simulink model "ACC_speed_change_curve_cs"  (R2016a)
settings: Solver=ode5  SolverMode=SingleTasking  StartTime=0.0  StopTime=inf  FixedStep=1/1000  RelTol=1e-3
PreLoadFcn:
  | mbxruntime.callbacks.PreLoadFcn(bdroot);
  | check_NUTS_defined;
  | 
  | assignin('base',['model_closed_' bdroot],false);addpath('../includes_ACC');
PostLoadFcn:
  | mbxruntime.callbacks.PostLoadFcn(bdroot);
InitFcn:
  | mbxruntime.callbacks.InitFcn(bdroot);
StartFcn:
  | mbxruntime.callbacks.StartFcn(bdroot);
StopFcn:
  | mbxruntime.callbacks.StopFcn(bdroot);
model workspace (MAT data in the model file):
  mbox_table : struct (value not decoded)
  model_closed = 0
  sim_status = 0
undefined symbols (not defined in the file or in its folder): DiscIntNeverNeededParam
undefined symbols (not defined in the file): SteeringColumn, SteeringWheel, WheelL0, WheelL1, WheelR0, WheelR1
libraries: simulink_extras x49, simulink x29, PreScanSimulinkLibrary x24, PreScanUsefulBlocks x2, Solver_SF x1, simulink_need_slupdate x1
(part 10 of 17)

== system ACC_speed_change_curve_cs/Audi_A8_1/ACC_System/TIS2 Straight Road ==
  note: === TIS2 Straight Road block ===
      |
      |  - interpretes information provided from the second TIS sensor,
      |  - computes HeadWay Time (HWT) for object on the lane in front of the EGO car,
      |  - determines if detected objects is potentially dengerous,
      |  - outputs distance to the following car, computes its velocity and safe distance to be kept.
  EGO_velocity [m/s] : Inport
  TIS2_range [m] : Inport  Port=2  PortDimensions=TISdet(2)
  TIS2_rangedot [m/s] : Inport  Port=3  PortDimensions=TISdet(2)
  TIS2_theta [deg] : Inport  Port=4  PortDimensions=TISdet(2)
  HWT_dem [s] : Inport  Port=5
  Standstill [m] : Inport  Port=6
  HWT_dem [s]1 : InportShadow  Port=5
  Hold : Subsystem
  TIS2 Closest Object : Subsystem
  TIS2 HWT Computing : Subsystem
  TIS2 HWT Computing2 : Subsystem
  TIS2 HWT Flag : Subsystem
  TIS2 Lead Car Longitudinal Velocity : Subsystem
  TIS2 Objects On Lane : Subsystem
  TIS2 Sorting Fun : Subsystem
  TIS2_closest_object_search : MATLAB Function  TreatAsAtomicUnit=on
  HWT_flag : Outport
  TIS2 Lead distance [m] : Outport  Port=2
  TIS2 Safe_distance [m] : Outport  Port=3
  TIS2_HWT_straight : Outport  Port=4
  TIS2 Lead velocity [m/s] : Outport  Port=5
  index : Outport  Port=6
  wires:
  TIS2 Lead Car Longitudinal Velocity/1(Safe distance [m]) -> TIS2 Safe_distance [m]/1
  HWT_dem [s]/1 -> TIS2 Lead Car Longitudinal Velocity/1(HWT_dem (s)), TIS2 HWT Flag/2(HWT_dem [s])
  TIS2 Closest Object/1(rangedot [m/s]) -> TIS2 Lead Car Longitudinal Velocity/2(TIS2 Rangedot [m/s])
  TIS2 Closest Object/2(distance [m/s]) -> TIS2 Lead distance [m]/1, TIS2 HWT Computing2/1(Distance [m]), TIS2 HWT Flag/1(Distance closest [m])
  EGO_velocity [m/s]/1 -> TIS2 Lead Car Longitudinal Velocity/3(EGO Velocity [m/s]), TIS2 HWT Computing2/2(Velocity [m/s]), TIS2 HWT Computing/3(Velocity [m/s])
  TIS2 HWT Computing/1(HWT [s]) -> TIS2 HWT Flag/3(HWT [s])
  TIS2_closest_object_search/1(index) -> TIS2 Closest Object/3(index), index/1
  TIS2 Sorting Fun/3(TIS2_THETA [rad]) -> TIS2 Objects On Lane/3(TIS2_theta [rad])
  TIS2 Sorting Fun/2(TIS2_RANGEDOT [m/s]) -> TIS2 Objects On Lane/2(TIS2_rangedot [m/s])
  TIS2 Sorting Fun/1(TIS2_RANGE [m]) -> TIS2 Objects On Lane/1(TIS2_range [m])
  TIS2_theta [deg]/1 -> TIS2 Sorting Fun/3(TIS2theta [deg])
  TIS2_rangedot [m/s]/1 -> TIS2 Sorting Fun/2(TIS2rangedot [m/s])
  TIS2_range [m]/1 -> TIS2 Sorting Fun/1(TIS2range [m])
  Standstill [m]/1 -> TIS2 Lead Car Longitudinal Velocity/4(Standstill [m]), TIS2 HWT Flag/4(Standstill distance)
  TIS2 Objects On Lane/1(TIS2_RANGEDOT [m/s]) -> TIS2 Closest Object/1(TIS2_rangedot [m/s])
  TIS2 Lead Car Longitudinal Velocity/2(Lead velocity [m/s]) -> TIS2 Lead velocity [m/s]/1, Hold/2(lead_vel_in)
  TIS2 HWT Computing2/1(HWT [s]) -> TIS2_HWT_straight/1
  TIS2 HWT Flag/1(HWT_flag) -> Hold/1(HWTflagIN)
  Hold/1(HWT_flag) -> HWT_flag/1
  HWT_dem [s]1/1 -> TIS2 HWT Computing/2(HWT demanded)
  TIS2 Objects On Lane/2(TIS2_Distance [m]) -> TIS2 Closest Object/2(TIS2_distance [m]), TIS2_closest_object_search/1(distance), TIS2 HWT Computing/1(Distance [m])

== system ACC_speed_change_curve_cs/Audi_A8_1/ACC_System3/Display ==
  HWT_% : Inport
  ACC_flag : Inport  Port=2
  Lead_car_velocity_[m/s] : Inport  Port=3
  RPM : Inport  Port=4
  EGO Velocity [m/s] : Inport  Port=5
  Brake_Pressure_[bar] : Inport  Port=6
  Throttle_[%] : Inport  Port=7
  Display switch : Constant  Value=DisplaySwitch
  If : If
  If Action Subsystem : Subsystem  TreatAsAtomicUnit=on
  If Action Subsystem1 : Subsystem  TreatAsAtomicUnit=on
  Merge : Merge  InitialOutput=1
  Rate Transition : RateTransition  Integrity=off  OutPortSampleTime=Tsensor
  Rate Transition{1..6,8} (7 alike) : RateTransition  Integrity=off  OutPortSampleTime=1/DisplayFreq
  "GUI_System ON {1} / OFF {0}" : Outport
  wires:
  Rate Transition/1 -> "GUI_System ON {1} / OFF {0}"/1
  Merge/1 -> Rate Transition/1
  If/2 -> If Action Subsystem1/Action
  If Action Subsystem1/1(Out1) -> Merge/2
  If Action Subsystem/1("GUI_System ON {1} / OFF {0}1") -> Merge/1
  If/1 -> If Action Subsystem/Action
  Rate Transition8/1 -> If Action Subsystem/7(Throttle_[%]1)
  Rate Transition6/1 -> If Action Subsystem/6(Lead_car_velocity_[m/s]1)
  Rate Transition5/1 -> If Action Subsystem/5(ACC_flag1)
  Rate Transition4/1 -> If Action Subsystem/4(HWT_%1)
  Rate Transition3/1 -> If Action Subsystem/3(Brake_Pressure_[bar]1)
  Rate Transition2/1 -> If Action Subsystem/2(EGO Velocity [m/s]1)
  Rate Transition1/1 -> If Action Subsystem/1(RPM1)
  Display switch/1 -> If/1
  Throttle_[%]/1 -> Rate Transition8/1
  Lead_car_velocity_[m/s]/1 -> Rate Transition6/1
  ACC_flag/1 -> Rate Transition5/1
  HWT_%/1 -> Rate Transition4/1
  Brake_Pressure_[bar]/1 -> Rate Transition3/1
  EGO Velocity [m/s]/1 -> Rate Transition2/1
  RPM/1 -> Rate Transition1/1

== system ACC_speed_change_curve_cs/Audi_A8_1/ACC_System3/HWT_percentage ==
  TIS1_HWT : Inport
  TIS2_HWT : Inport  Port=2  SampleTime=Tsensor
  HWT_dem_[s] : Inport  Port=3  SampleTime=Tsensor
  Bias : Bias  Bias=-1
  Brake Pressure [ar]1 : Gain  Gain=100
  Constant : Constant  Value=10
  Constant1 : Constant  Value=0
  Demux : Demux  Outputs=2
  Divide : Product  Inputs=*/
  Logical Operator : Logic  AllPortsSameDT=off  OutDataTypeStr=boolean
  Mux : Mux  Inputs=2
  Relational Operator : RelationalOperator  Operator=<  OutDataTypeStr=boolean
  Relational Operator1 : RelationalOperator  Operator=>  OutDataTypeStr=boolean
  TIS1_HWT_perc : Outport
  TIS2_HWT_perc : Outport  Port=2
  wires:
  Constant1/1 -> Relational Operator1/2
  Relational Operator1/1 -> Logical Operator/2
  Logical Operator/1 -> Demux/1
  Relational Operator/1 -> Logical Operator/1
  Demux/2 -> TIS2_HWT_perc/1
  Demux/1 -> TIS1_HWT_perc/1
  HWT_dem_[s]/1 -> Divide/2
  Mux/1 -> Relational Operator1/1, Divide/1
  Constant/1 -> Relational Operator/2
  Brake Pressure [ar]1/1 -> Relational Operator/1
  TIS2_HWT/1 -> Mux/2
  TIS1_HWT/1 -> Mux/1
  Bias/1 -> Brake Pressure [ar]1/1
  Divide/1 -> Bias/1

== system ACC_speed_change_curve_cs/Audi_A8_1/ACC_System3/Limitations1 ==
  note: === Limitations block ===
      |
      |  - switching the system on or off due to the drivers decision,
      |  - limits maximum operating velocity
      |    above which the sensors are becoming ineffective.
  note: if equal to 1 => ACC should be off
      | if equal to 0 => ACC should be on
  Throttle [%] : Inport
  Brake_Pres [bar] : Inport  Port=2
  ACC_flag : Inport  Port=3
  HWT [s] : Inport  Port=4
  Lead car vel : Inport  Port=5
  indx : Inport  Port=6
  "Switch ON {1} / OFF {0}" : Inport  Port=7
  EGO Velocity [m/s] : Inport  Port=8
  Indicator flag : Inport  Port=9
  Throttle_in [%] : Inport  Port=10
  Brake_Pres_in [bar] : Inport  Port=11
  HWT_dem_[s] : Inport  Port=12
  TIS2_Flag : Inport  Port=13
  Compare To Zero : simulink/Logic and Bit Operations/Compare To Zero  relop===  OutDataTypeStr=boolean
  Compare To Zero1 : simulink/Logic and Bit Operations/Compare To Zero  relop=~=  OutDataTypeStr=boolean
  Const : Constant  Value=BrakePressureMax/100
  Constant : Constant  Value=TISdet (2)
  Constant1 : Constant  Value=TISdet (1)
  Gain : Gain  Gain=2
  Gain1 : Gain
  Gain2 : Gain
  Logical Operator : Logic  Operator=OR  Inputs=3  AllPortsSameDT=off  OutDataTypeStr=boolean
  Logical Operator1 : Logic  Operator=OR  AllPortsSameDT=off  OutDataTypeStr=boolean
  MAX Speed [m/s] : Constant  Value=MaxSpeed/3.6
  Rate Limiter : RateLimiter  RisingSlewLimit=BrakePressureMax  FallingSlewLimit=-BrakePressureMax  SampleTimeMode=inherited
  Rate Transition : RateTransition  Integrity=off  OutPortSampleTime=Tsensor
  Relational Operator : RelationalOperator  Operator=>  OutDataTypeStr=boolean
  Relational Operator1 : RelationalOperator  OutDataTypeStr=boolean
  Relational Operator2 : RelationalOperator  Operator===  OutDataTypeStr=boolean
  Saturation Dynamic : simulink/Discontinuities/Saturation Dynamic  OutMin=[]  OutMax=[]  OutDataTypeStr=Inherit: Same as second input  OutDataType=fixdt(1, 16)  OutScaling=2^-10  DoSatur=off
  Switch{,1..6} (7 alike) : Switch  Criteria=u2 > Threshold
  Switch7 : Switch  Criteria=u2 ~= 0
  Zero : Constant  Value=0
  Zero1 : Constant  Value=0
  cond : Subsystem
  Throttle_out [%] : Outport
  Brake_Pres_out [bar] : Outport  Port=2
  ACC flag : Outport  Port=3
  HWT_[s] : Outport  Port=4
  Lead car velocity [m/s] : Outport  Port=5
  wires:
  Rate Limiter/1 -> Switch7/1
  Switch/1 -> Rate Limiter/1, Switch7/3
  Switch7/1 -> Switch4/1, Relational Operator1/1
  cond/1(Out1) -> Switch7/2
  Brake_Pres [bar]/1 -> Switch/3
  Brake_Pres_in [bar]/1 -> Switch/1
  Relational Operator2/1 -> Logical Operator1/2
  Constant1/1 -> Switch6/3
  Constant/1 -> Switch6/1
  Switch6/1 -> Relational Operator2/1
  TIS2_Flag/1 -> Switch6/2
  Rate Transition/1 -> Logical Operator1/1
  Switch4/1 -> Brake_Pres_out [bar]/1
  Zero1/1 -> Switch4/3
  Relational Operator1/1 -> Switch4/2
  Const/1 -> Relational Operator1/2
  Saturation Dynamic/1 -> HWT_[s]/1
  Switch3/1 -> Saturation Dynamic/2
  HWT [s]/1 -> Switch3/3
  Logical Operator1/1 -> Switch3/2
  indx/1 -> Relational Operator2/2
  Lead car vel/1 -> Switch5/3
  Switch5/1 -> Lead car velocity [m/s]/1
  Gain2/1 -> Compare To Zero1/1
  Gain1/1 -> Compare To Zero/1
  Gain/1 -> Saturation Dynamic/1
  HWT_dem_[s]/1 -> Gain/1
  Compare To Zero1/1 -> Logical Operator/3
  Relational Operator/1 -> Logical Operator/2
  Compare To Zero/1 -> Logical Operator/1
  Switch2/1 -> ACC flag/1
  Switch1/1 -> Throttle_out [%]/1
  ACC_flag/1 -> Switch2/3
  Throttle [%]/1 -> Switch1/3
  Zero/1 -> Saturation Dynamic/3, Switch3/1, Switch5/1, Switch2/1
  Throttle_in [%]/1 -> Switch1/1
  Logical Operator/1 -> Switch/2, Rate Transition/1, Switch5/2, Switch2/2, Switch1/2, cond/1(In1)
  Indicator flag/1 -> Gain2/1
  "Switch ON {1} / OFF {0}"/1 -> Gain1/1
  MAX Speed [m/s]/1 -> Relational Operator/2
  EGO Velocity [m/s]/1 -> Relational Operator/1

== system ACC_speed_change_curve_cs/Audi_A8_1/ACC_System3/Limitations2 ==
  Throttle [%] : Inport
  Brake_Pres [bar] : Inport  Port=2
  ACC_flag : Inport  Port=3
  HWT [s] : Inport  Port=4
  Lead car vel : Inport  Port=5
  "Switch ON {1} / OFF {0}" : Inport  Port=6
  Throttle_in [%] : Inport  Port=7
  Brake_Pres_in [bar] : Inport  Port=8
  ACC_flag1 : InportShadow  Port=3
  Brake_Pres_in [bar]1 : InportShadow  Port=8
  Constant : Constant  Value=[0;0;0]
  Demux : Demux  Outputs=5
  Gain : Gain  Gain=3.6
  Lead car vel1 : InportShadow  Port=5
  Logical Operator : Logic  Operator=OR  AllPortsSameDT=off  OutDataTypeStr=boolean
  LowActiv : Constant  Value=LowSpeedActv
  Mux1 : Mux  Inputs=3
  Mux2 : Mux  Inputs=5
  Mux3 : Mux  Inputs=5
  Rate Limiter : RateLimiter  RisingSlewLimit=BrakeMax*1e3  FallingSlewLimit=-BrakeMax*1e3  SampleTimeMode=inherited
  Relational Operator1 : RelationalOperator  Operator=>  OutDataTypeStr=boolean
  Saturation : Saturate  UpperLimit=BrakePressureMax  LowerLimit=0
  Switch : Switch  Criteria=u2 ~= 0
  Switch1 : Switch  Criteria=u2 ~= 0
  Throttle_in [%]1 : InportShadow  Port=7
  cond1 : Subsystem
  Throttle_out [%] : Outport
  Brake_Pres_out [bar] : Outport  Port=2
  HWT_[s] : Outport  Port=3
  ACC flag : Outport  Port=4
  Lead car velocity [m/s] : Outport  Port=5
  wires:
  cond1/1(Out1) -> Switch/2
  Relational Operator1/1 -> Logical Operator/2
  ACC_flag1/1 -> Logical Operator/1
  Logical Operator/1 -> Switch1/2
  Lead car vel1/1 -> Gain/1
  Gain/1 -> Relational Operator1/2
  LowActiv/1 -> Relational Operator1/1
  Brake_Pres_in [bar]1/1 -> Saturation/1
  Throttle_in [%]1/1 -> Rate Limiter/1
  Demux/5 -> Lead car velocity [m/s]/1
  Demux/4 -> ACC flag/1
  Demux/3 -> HWT_[s]/1
  Demux/2 -> Brake_Pres_out [bar]/1
  Demux/1 -> Throttle_out [%]/1
  Switch/1 -> Demux/1
  Switch1/1 -> Switch/1
  Mux3/1 -> Switch1/3
  Saturation/1 -> Mux3/2
  Rate Limiter/1 -> Mux3/1
  Mux2/1 -> Switch1/1
  Lead car vel/1 -> Mux3/5, Mux2/5
  ACC_flag/1 -> Mux3/4, Mux2/4
  HWT [s]/1 -> Mux3/3, Mux2/3
  Brake_Pres [bar]/1 -> Mux2/2
  Throttle [%]/1 -> Mux2/1
  Mux1/1 -> Switch/3
  Constant/1 -> Mux1/3
  Brake_Pres_in [bar]/1 -> Mux1/2
  Throttle_in [%]/1 -> Mux1/1
  "Switch ON {1} / OFF {0}"/1 -> cond1/1(In1)

== system ACC_speed_change_curve_cs/Audi_A8_1/ACC_System3/Radar ==
  TIS1 Range : Inport
  TIS1 Theta : Inport  Port=2
  TIS2 Range : Inport  Port=3
  TIS2 Theta : Inport  Port=4
  TIS1_index : Inport  Port=5
  TIS2_index : Inport  Port=6
  TIS1_HWT_% : Inport  Port=7
  TIS2_HWT_% : Inport  Port=8
  System switch : Inport  Port=9
  Radar : Subsystem
  Radar switch : Constant  Value=RadarSwitch
  Rate Transition{1..6,8..10} (9 alike) : RateTransition  Integrity=off  OutPortSampleTime=1/RadarFreq
  wires:
  Rate Transition6/1 -> Radar/9(System switch)
  System switch/1 -> Rate Transition6/1
  Rate Transition4/1 -> Radar/6(TIS2_index)
  TIS2_index/1 -> Rate Transition4/1
  Rate Transition10/1 -> Radar/8(TIS2_HWT_%)
  Rate Transition9/1 -> Radar/7(TIS1_HWT_%)
  TIS2_HWT_%/1 -> Rate Transition10/1
  TIS1_HWT_%/1 -> Rate Transition9/1
  TIS1_index/1 -> Rate Transition8/1
  Rate Transition8/1 -> Radar/5(TIS1_index)
  Radar switch/1 -> Radar/Enable
  Rate Transition3/1 -> Radar/4(TIS2 Theta)
  Rate Transition2/1 -> Radar/3(TIS2 Range)
  Rate Transition1/1 -> Radar/2(TIS1 Theta)
  Rate Transition5/1 -> Radar/1(TIS1 Range)
  TIS2 Theta/1 -> Rate Transition3/1
  TIS2 Range/1 -> Rate Transition2/1
  TIS1 Theta/1 -> Rate Transition1/1
  TIS1 Range/1 -> Rate Transition5/1

== system ACC_speed_change_curve_cs/Audi_A8_1/ACC_System3/Rate transition from other signals ==
  In1 : Inport
  In2 : Inport  Port=2
  Rate Transition1 : RateTransition  Integrity=off  OutPortSampleTime=Tsensor
  Rate Transition2 : RateTransition  Integrity=off  OutPortSampleTime=Tsensor
  Out1 : Outport
  Out2 : Outport  Port=2
  wires:
  In1/1 -> Rate Transition1/1
  Rate Transition1/1 -> Out1/1
  In2/1 -> Rate Transition2/1
  Rate Transition2/1 -> Out2/1

== system ACC_speed_change_curve_cs/Audi_A8_1/ACC_System3/Rate transition from EGO ==
  In1 : Inport
  In2 : Inport  Port=2
  In3 : Inport  Port=3
  In4 : Inport  Port=4
  In5 : Inport  Port=5
  In6 : Inport  Port=6
  Rate Transition{1..6} (6 alike) : RateTransition  Integrity=off  OutPortSampleTime=Tsensor
  Out1 : Outport
  Out2 : Outport  Port=2
  Out3 : Outport  Port=3
  Out4 : Outport  Port=4
  Out5 : Outport  Port=5
  Out6 : Outport  Port=6
  wires:
  Rate Transition6/1 -> Out6/1
  In6/1 -> Rate Transition6/1
  Rate Transition5/1 -> Out5/1
  In5/1 -> Rate Transition5/1
  Rate Transition4/1 -> Out4/1
  In4/1 -> Rate Transition4/1
  Rate Transition3/1 -> Out3/1
  In3/1 -> Rate Transition3/1
  Rate Transition2/1 -> Out2/1
  In2/1 -> Rate Transition2/1
  Rate Transition1/1 -> Out1/1
  In1/1 -> Rate Transition1/1

== system ACC_speed_change_curve_cs/Audi_A8_1/ACC_System3/Rate transition from TIS1 ==
  In1 : Inport
  In2 : Inport  Port=2
  In3 : Inport  Port=3
  Rate Transition1 : RateTransition  Integrity=off  OutPortSampleTime=Tsensor
  Rate Transition2 : RateTransition  Integrity=off  OutPortSampleTime=Tsensor
  Rate Transition3 : RateTransition  Integrity=off  OutPortSampleTime=Tsensor
  Out1 : Outport
  Out2 : Outport  Port=2
  Out3 : Outport  Port=3
  wires:
  In1/1 -> Rate Transition1/1
  Rate Transition1/1 -> Out1/1
  In2/1 -> Rate Transition2/1
  Rate Transition2/1 -> Out2/1
  In3/1 -> Rate Transition3/1
  Rate Transition3/1 -> Out3/1

== system ACC_speed_change_curve_cs/Audi_A8_1/ACC_System3/Rate transition from TIS2 ==
  In1 : Inport
  In2 : Inport  Port=2
  In3 : Inport  Port=3
  Rate Transition1 : RateTransition  Integrity=off  OutPortSampleTime=Tsensor
  Rate Transition2 : RateTransition  Integrity=off  OutPortSampleTime=Tsensor
  Rate Transition3 : RateTransition  Integrity=off  OutPortSampleTime=Tsensor
  Out1 : Outport
  Out2 : Outport  Port=2
  Out3 : Outport  Port=3
  wires:
  Rate Transition2/1 -> Out3/1
  In3/1 -> Rate Transition2/1
  Rate Transition1/1 -> Out2/1
  In2/1 -> Rate Transition1/1
  Rate Transition3/1 -> Out1/1
  In1/1 -> Rate Transition3/1

== system ACC_speed_change_curve_cs/Audi_A8_1/ACC_System3/Sensors data merge ==
  note: === Sensors data merge block ===
      |
      |  - merges data from both sensors,
      |  - chooses the second, short - range sensor as major,
      |  - limits acceleration and deceleration of the EGO car.
  TIS1_Flag : Inport
  TIS1_Throttle [%] : Inport  Port=2
  TIS1_BrakePres [bar] : Inport  Port=3
  TIS1_HWT : Inport  Port=4
  TIS1_lead_velocity : Inport  Port=5
  TIS1_indx : Inport  Port=6
  TIS2_Flag : Inport  Port=7
  TIS2_Throttle [%] : Inport  Port=8
  TIS2_BrakePres [bar] : Inport  Port=9
  TIS2_HWT : Inport  Port=10
  TIS2_lead_velocity : Inport  Port=11
  TIS2_indx : Inport  Port=12
  Rate Limiter : RateLimiter  RisingSlewLimit=16  FallingSlewLimit=-inf  SampleTimeMode=inherited
  Saturation : Saturate  UpperLimit=100  LowerLimit=0
  Saturation1 : Saturate  UpperLimit=BrakePressureMax  LowerLimit=0
  Switch{,1,3..6} (6 alike) : Switch  Criteria=u2 > Threshold
  Switch2 : Switch  Criteria=u2 ~= 0
  Throttle_out [%] : Outport
  BrakePres_out [bar] : Outport  Port=2
  ACC_flag : Outport  Port=3
  HWT [s] : Outport  Port=4
  Lead_car_velocity : Outport  Port=5
  indx : Outport  Port=6
  wires:
  Switch5/1 -> indx/1
  TIS1_indx/1 -> Switch5/3
  TIS2_indx/1 -> Switch5/1
  Switch6/1 -> Lead_car_velocity/1
  TIS1_lead_velocity/1 -> Switch6/3
  TIS2_lead_velocity/1 -> Switch6/1
  Saturation1/1 -> BrakePres_out [bar]/1
  TIS1_HWT/1 -> Switch4/3
  TIS2_HWT/1 -> Switch4/1
  Switch4/1 -> HWT [s]/1
  Switch3/1 -> ACC_flag/1
  TIS1_Flag/1 -> Switch3/3
  Rate Limiter/1 -> Switch2/3
  Saturation/1 -> Rate Limiter/1, Switch2/1
  Switch2/1 -> Throttle_out [%]/1
  Switch1/1 -> Switch2/2, Saturation1/1
  Switch/1 -> Saturation/1
  TIS1_BrakePres [bar]/1 -> Switch1/3
  TIS1_Throttle [%]/1 -> Switch/3
  TIS2_BrakePres [bar]/1 -> Switch1/1
  TIS2_Throttle [%]/1 -> Switch/1
  TIS2_Flag/1 -> Switch5/2, Switch6/2, Switch4/2, Switch3/2, Switch3/1, Switch1/2, Switch/2

== system ACC_speed_change_curve_cs/Audi_A8_1/ACC_System3/Switching TIS ==
  note: === Switching block ===
      |
      |  - determines if the EGO car is moving on a straight road or on a bend raod,
      |  - based on the actual value of the yaw rate of the EGO car.
  straight_mux : Inport
  EGO_Yaw_rate_[deg/s] : Inport  Port=2
  bend_mux : Inport  Port=3
  1deg_per_s : Constant
  Abs : Abs
  Relational Operator : RelationalOperator  Operator=<  OutDataTypeStr=boolean
  Selector : Selector  InputPortWidth=12  IndexOptions=Index vector (dialog)  Indices=[6 12]  OutputSizes=1
  Switch : Switch  Criteria=u2 ~= 0  Threshold=0.5
  demux : Outport
  indexes : Outport  Port=2
  wires:
  Selector/1 -> indexes/1
  Abs/1 -> Relational Operator/1
  bend_mux/1 -> Switch/3
  Switch/1 -> Selector/1, demux/1
  straight_mux/1 -> Switch/1
  Relational Operator/1 -> Switch/2
  1deg_per_s/1 -> Relational Operator/2
  EGO_Yaw_rate_[deg/s]/1 -> Abs/1

== system ACC_speed_change_curve_cs/Audi_A8_1/ACC_System3/TIS1 ACC action ==
  note: === TIS1 ACC action block ===
      |
      |  - control block,
      |  - uses information provided by the first sensor,
      |  - limits acceleration and deceleration of the EGO car,
      |  - adjusts throttle and brake pressure of the EGO car,
      |  - the control strategy is to maintain HeadWay Time (HWT)
      |    on desirable level.
  EGO Velocity [m/s] : Inport
  th_in [%] : Inport  Port=2
  br_in [bar] : Inport  Port=3
  HWT_demanded_[s] : Inport  Port=4
  TIS1_HWT_flag : Inport  Port=5
  TIS1_distance [m] : Inport  Port=6
  TIS1_safe_distance [m] : Inport  Port=7
  TIS1_HWT : Inport  Port=8
  TIS1_lead_velocity_[m/s] : Inport  Port=9
  indx : Inport  Port=10
  Add : Sum  Inputs=+-
  Add1 : Sum  Inputs=+-
  Add2 : Sum  Inputs=+-
  Gain : Gain
  Gain1 : Gain  Gain=J_xx/Qfac/Rw
  Gain2 : Gain
  HWT_demanded_[s]1 : InportShadow  Port=4
  HWT_demanded_[s]2 : InportShadow  Port=4
  If : If  IfExpression=u1 >= 0  SampleTime=Tsensor
  If Action Subsystem : Subsystem  TreatAsAtomicUnit=on
  If Action Subsystem1 : Subsystem  TreatAsAtomicUnit=on
  Merge : Merge
  Merge1 : Merge
  Rate Limiter : RateLimiter  RisingSlewLimit=BrakeMax  FallingSlewLimit=-BrakeMax  SampleTimeMode=inherited
  Saturation : Saturate  UpperLimit=BrakeMax  LowerLimit=0
  Switch : Switch  Criteria=u2 > Threshold
  Switch1 : Switch  Criteria=u2 > Threshold
  TIS1_distance [m]1 : InportShadow  Port=6
  TIS1_distance [m]2 : InportShadow  Port=6
  TIS1_lead_velocity_[m/s]1 : InportShadow  Port=9
  TIS1_lead_velocity_[m/s]2 : InportShadow  Port=9
  th_in [%]1 : InportShadow  Port=2
  TIS1_flag : Outport
  throttle : Outport  Port=2
  TIS1_br_out [bar] : Outport  Port=3
  TIS1_HWTo : Outport  Port=4
  TIS1_Lead_velocity_[m/s] : Outport  Port=5
  indx2 : Outport  Port=6
  wires:
  Rate Limiter/1 -> Gain1/1
  indx/1 -> indx2/1
  th_in [%]1/1 -> If Action Subsystem/6(th in)
  HWT_demanded_[s]2/1 -> If Action Subsystem/5(HWT dem)
  TIS1_distance [m]2/1 -> If Action Subsystem/4(EGO distance)
  TIS1_lead_velocity_[m/s]2/1 -> If Action Subsystem/3(Vp)
  HWT_demanded_[s]1/1 -> If Action Subsystem1/5(HWT dem)
  TIS1_lead_velocity_[m/s]1/1 -> If Action Subsystem1/3(Vp)
  TIS1_distance [m]1/1 -> If Action Subsystem1/4(EGO dis)
  th_in [%]/1 -> Switch1/3
  br_in [bar]/1 -> Switch/3
  Merge1/1 -> Switch1/1
  Gain1/1 -> Switch/1
  Switch1/1 -> Gain2/1
  Switch/1 -> Gain/1
  TIS1_HWT_flag/1 -> Switch/2, Switch1/2, TIS1_flag/1
  Merge/1 -> Saturation/1
  Saturation/1 -> Rate Limiter/1
  If Action Subsystem1/2(throttle) -> Merge1/2
  If Action Subsystem/2(throttle) -> Merge1/1
  If Action Subsystem1/1(dec) -> Merge/2
  If Action Subsystem/1(dec) -> Merge/1
  Add2/1 -> If Action Subsystem/2(e), If Action Subsystem1/2(e)
  TIS1_safe_distance [m]/1 -> Add2/2
  TIS1_distance [m]/1 -> Add2/1
  Add1/1 -> If Action Subsystem1/1(rd), If Action Subsystem/1(rd)
  TIS1_lead_velocity_[m/s]/1 -> TIS1_Lead_velocity_[m/s]/1, Add1/2
  EGO Velocity [m/s]/1 -> Add1/1
  If/2 -> If Action Subsystem1/Action
  If/1 -> If Action Subsystem/Action
  Add/1 -> If/1
  HWT_demanded_[s]/1 -> Add/2
  TIS1_HWT/1 -> TIS1_HWTo/1, Add/1
  Gain/1 -> TIS1_br_out [bar]/1
  Gain2/1 -> throttle/1

== system ACC_speed_change_curve_cs/Audi_A8_1/ACC_System3/TIS1 Bend Road ==
  note: === TIS1 Bend Road block ===
      |
      |  - interpretes information provided from the first TIS sensor,
      |  - computes HeadWay Time (HWT) for object on the lane of the EGO car on the bend road,
      |  - determines if detected objects is potentially dengerous,
      |  - outputs distance to the following car, computes its velocity and safe distance to be kept.
  EGO_velocity [m/s] : Inport
  TIS1_range [m] : Inport  Port=2  PortDimensions=TISdet(1)
  TIS1_rangedot [m/s] : Inport  Port=3  PortDimensions=TISdet(1)
  TIS1_theta [deg] : Inport  Port=4  PortDimensions=TISdet(1)
  HWT_dem [s] : Inport  Port=5
  Standstill [m] : Inport  Port=6
  EGO_Yaw_rate [deg/s] : Inport  Port=7
  EGO_velocity [m/s]2 : InportShadow
  Embedded MATLAB Function : MATLAB Function  TreatAsAtomicUnit=on
  Hold : Subsystem
  Lead Car Longitudinal Velocity : Subsystem
  TIS1 Closest Object On Bend Road : Subsystem
  TIS1 HWT Computing : Subsystem
  TIS1 HWT Flag : Subsystem
  TIS1 Objects On Bend Road : Subsystem
  TIS1 Sorting  Fun : Subsystem
  HWT_flag : Outport
  TIS1 Lead distance [m] : Outport  Port=2
  TIS1 Safe_distance [m] : Outport  Port=3
  TIS1_HWT_bend : Outport  Port=4
  TIS1 lead velocity [m/s] : Outport  Port=5
  index : Outport  Port=6
  wires:
  TIS1 Closest Object On Bend Road/1(range [m]) -> Lead Car Longitudinal Velocity/7(TIS1 Range [m])
  TIS1 HWT Flag/1(HWT_flag) -> Hold/1(HWTflagIN)
  Hold/1(HWT_flag) -> HWT_flag/1
  Lead Car Longitudinal Velocity/2(Lead velocity [m/s]) -> Hold/2(lead_vel_in), TIS1 lead velocity [m/s]/1
  Lead Car Longitudinal Velocity/1(Safe distance [m]) -> TIS1 Safe_distance [m]/1
  TIS1 Closest Object On Bend Road/5(lambda [rad]) -> Lead Car Longitudinal Velocity/6(lambda [rad])
  TIS1 Closest Object On Bend Road/3(theta [rad]) -> Lead Car Longitudinal Velocity/5(theta [rad])
  Standstill [m]/1 -> TIS1 HWT Flag/4(Standstill distance), Lead Car Longitudinal Velocity/4(Standstill [m])
  HWT_dem [s]/1 -> TIS1 HWT Flag/3(HWT_dem [s]), Lead Car Longitudinal Velocity/1(HWT_dem (s))
  TIS1 HWT Computing/1(HWT [s]) -> TIS1 HWT Flag/2(HWT [s]), TIS1_HWT_bend/1
  TIS1 Closest Object On Bend Road/2(rangedot [m/s]) -> Lead Car Longitudinal Velocity/2(TIS1 Rangedot [m/s])
  EGO_velocity [m/s]2/1 -> TIS1 HWT Computing/2(Velocity [m/s]), Lead Car Longitudinal Velocity/3(EGO Velocity [m/s])
  TIS1 Closest Object On Bend Road/4(Distance [m]) -> TIS1 HWT Flag/1(Distance closest [m]), TIS1 HWT Computing/1(Distance [m]), TIS1 Lead distance [m]/1
  TIS1 Objects On Bend Road/5(TIS1_lambda_[rad]) -> TIS1 Closest Object On Bend Road/6(TIS1_lambda [rad])
  TIS1 Objects On Bend Road/4(TIS1_Distance [m]) -> TIS1 Closest Object On Bend Road/5(TIS1_Distance [m])
  TIS1 Objects On Bend Road/3(TIS1_THETA [rad]) -> TIS1 Closest Object On Bend Road/4(TIS1_theta [rad])
  TIS1 Objects On Bend Road/2(TIS1_RANGEDOT [m/s]) -> TIS1 Closest Object On Bend Road/3(TIS1_rangedot [m])
  TIS1 Objects On Bend Road/1(TIS1_RANGE [m]) -> Embedded MATLAB Function/1(distance), TIS1 Closest Object On Bend Road/2(TIS1_range [m])
  Embedded MATLAB Function/1(index) -> index/1, TIS1 Closest Object On Bend Road/1(index)
  EGO_Yaw_rate [deg/s]/1 -> TIS1 Objects On Bend Road/5(EGO_Yaw_rate_[deg/s])
  EGO_velocity [m/s]/1 -> TIS1 Objects On Bend Road/4(EGO_Velocity [m/s])
  TIS1 Sorting  Fun/3(TIS1_THETA [rad]) -> TIS1 Objects On Bend Road/3(TIS1_theta [rad])
  TIS1 Sorting  Fun/2(TIS1_RANGEDOT [m/s]) -> TIS1 Objects On Bend Road/2(TIS1_rangedot [m/s])
  TIS1 Sorting  Fun/1(TIS1_RANGE [m]) -> TIS1 Objects On Bend Road/1(TIS1_range [m])
  TIS1_range [m]/1 -> TIS1 Sorting  Fun/1(TIS1range [m])
  TIS1_rangedot [m/s]/1 -> TIS1 Sorting  Fun/2(TIS1rangedot [m/s])
  TIS1_theta [deg]/1 -> TIS1 Sorting  Fun/3(TIS1theta [deg])

== system ACC_speed_change_curve_cs/Audi_A8_1/ACC_System3/TIS1 Straight Road ==
  note: === TIS1 Straight Road block ===
      |
      |  - interpretes information provided from the first TIS sensor,
      |  - computes HeadWay Time (HWT) for object on the lane in front of the EGO car,
      |  - determines if detected objects is potentially dengerous,
      |  - outputs distance to the following car, computes its velocity and safe distance to be kept.
  EGO_velocity [m/s] : Inport
  TIS1_range [m] : Inport  Port=2  PortDimensions=TISdet(1)
  TIS1_rangedot [m/s] : Inport  Port=3  PortDimensions=TISdet(1)
  TIS1_theta [deg] : Inport  Port=4  PortDimensions=TISdet(1)
  HWT_dem [s] : Inport  Port=5
  Standstill [m] : Inport  Port=6
  HWT_dem [s]1 : InportShadow  Port=5
  Hold : Subsystem
  TIS1 Closest Object : Subsystem
  TIS1 HWT Computing : Subsystem
  TIS1 HWT Computing1 : Subsystem
  TIS1 HWT Flag : Subsystem
  TIS1 Lead Car Longitudinal Velocity : Subsystem
  TIS1 Objects On Lane : Subsystem
  TIS1 Sorting Fun : Subsystem
  TIS1_closest_object_search : MATLAB Function  TreatAsAtomicUnit=on
  HWT_flag : Outport
  TIS1 Lead distance [m] : Outport  Port=2
  TIS1 Safe_distance [m] : Outport  Port=3
  TIS1_HWT_straight : Outport  Port=4
  TIS1 Lead velocity [m/s] : Outport  Port=5
  index : Outport  Port=6
  wires:
  TIS1 Objects On Lane/2(TIS1_Distance [m]) -> TIS1_closest_object_search/1(distance), TIS1 HWT Computing/1(Distance [m]), TIS1 Closest Object/2(TIS1_Distance [m])
  Hold/1(HWT_flag) -> HWT_flag/1
  TIS1 Lead Car Longitudinal Velocity/2(Safe distance [m]) -> TIS1 Safe_distance [m]/1
  TIS1 Lead Car Longitudinal Velocity/1(lead_velocity [m/s]) -> TIS1 Lead velocity [m/s]/1, Hold/2(lead_vel_in)
  TIS1 HWT Flag/1(HWT_flag) -> Hold/1(HWTflagIN)
  TIS1 HWT Computing1/1(HWT [s]) -> TIS1_HWT_straight/1
  HWT_dem [s]1/1 -> TIS1 HWT Computing/2(HWT demanded)
  TIS1 Closest Object/2(Distance [m/s]) -> TIS1 HWT Flag/1(Distance closest [m]), TIS1 HWT Computing1/1(Distance [m]), TIS1 Lead distance [m]/1
  TIS1 Closest Object/1(rangedot [m/s]) -> TIS1 Lead Car Longitudinal Velocity/2(TIS1 Rangedot [m/s])
  EGO_velocity [m/s]/1 -> TIS1 HWT Computing/3(Velocity [m/s]), TIS1 HWT Computing1/2(Velocity [m/s]), TIS1 Lead Car Longitudinal Velocity/3(EGO Velocity [m/s])
  Standstill [m]/1 -> TIS1 HWT Flag/4(Standstill distance), TIS1 Lead Car Longitudinal Velocity/4(Standstill [m])
  TIS1 Objects On Lane/1(TIS1_RANGEDOT [m/s]) -> TIS1 Closest Object/1(TIS1_rangedot [m/s])
  HWT_dem [s]/1 -> TIS1 HWT Flag/2(HWT_dem [s]), TIS1 Lead Car Longitudinal Velocity/1(HWT_dem (s))
  TIS1 HWT Computing/1(HWT [s]) -> TIS1 HWT Flag/3(HWT [s])
  TIS1_closest_object_search/1(index) -> index/1, TIS1 Closest Object/3(index)
  TIS1 Sorting Fun/3(TIS1_THETA [rad]) -> TIS1 Objects On Lane/3(TIS1_theta [rad])
  TIS1 Sorting Fun/2(TIS1_RANGEDOT [m/s]) -> TIS1 Objects On Lane/2(TIS1_rangedot [m/s])
  TIS1 Sorting Fun/1(TIS1_RANGE [m]) -> TIS1 Objects On Lane/1(TIS1_range [m])
  TIS1_theta [deg]/1 -> TIS1 Sorting Fun/3(TIS1theta [deg])
  TIS1_rangedot [m/s]/1 -> TIS1 Sorting Fun/2(TIS1rangedot [m/s])
  TIS1_range [m]/1 -> TIS1 Sorting Fun/1(TIS1range [m])

== system ACC_speed_change_curve_cs/Audi_A8_1/ACC_System3/TIS2 ACC action ==
  note: === TIS2 ACC action block ===
      |
      |  - control block,
      |  - uses information provided by the second sensor,
      |  - limits acceleration and deceleration of the EGO car,
      |  - adjusts throttle and brake pressure of the EGO car,
      |  - the control strategy is to maintain HeadWay Time (HWT)
      |    on desirable level.
  TIS2_HWT_flag : Inport
  TIS2_distance [m] : Inport  Port=2
  TIS2_safe_distance [m] : Inport  Port=3
  TIS2_HWT : Inport  Port=4
  TIS2_lead_velocity_[m/s] : Inport  Port=5
  indx : Inport  Port=6
  th_in [%] : Inport  Port=7
  br_in [bar] : Inport  Port=8
  HWT_demanded_[s] : Inport  Port=9
  EGO Velocity [m/s] : Inport  Port=10
  Stand : Inport  Port=11
  Add : Sum  Inputs=+-
  Add1 : Sum  Inputs=+-
  Add2 : Sum  Inputs=+-
  EGO Velocity [m/s]1 : InportShadow  Port=10
  Gain1 : Gain  Gain=J_xx/Qfac/Rw
  HWT_demanded_[s]1 : InportShadow  Port=9
  HWT_demanded_[s]2 : InportShadow  Port=9
  If : If  IfExpression=u1 >= 0
  If Action Subsystem : Subsystem  TreatAsAtomicUnit=on
  If Action Subsystem1 : Subsystem  TreatAsAtomicUnit=on
  Merge : Merge
  Merge1 : Merge
  Rate Limiter : RateLimiter  RisingSlewLimit=BrakeRateMax  FallingSlewLimit=-BrakeRateMax  SampleTimeMode=inherited
  Saturation : Saturate  UpperLimit=BrakeMax  LowerLimit=0
  Stop & Go : Subsystem
  Switch : Switch  Criteria=u2 > Threshold
  Switch1 : Switch  Criteria=u2 > Threshold
  TIS2_distance [m]1 : InportShadow  Port=2
  TIS2_distance [m]2 : InportShadow  Port=2
  TIS2_distance [m]3 : InportShadow  Port=2
  TIS2_lead_velocity_[m/s]1 : InportShadow  Port=5
  TIS2_lead_velocity_[m/s]2 : InportShadow  Port=5
  TIS2_safe_distance [m]1 : InportShadow  Port=3
  th_in [%]1 : InportShadow  Port=7
  TIS2_flag : Outport
  TIS2_th_out [%] : Outport  Port=2
  TIS2_br_out [bar] : Outport  Port=3
  TIS2_HWTo : Outport  Port=4
  TIS2_Lead_velocity_[m/s] : Outport  Port=5
  indx2 : Outport  Port=6
  wires:
  Rate Limiter/1 -> Gain1/1
  indx/1 -> indx2/1
  TIS2_lead_velocity_[m/s]2/1 -> If Action Subsystem/3(Vp)
  TIS2_distance [m]2/1 -> If Action Subsystem/4(EGO distance)
  HWT_demanded_[s]2/1 -> If Action Subsystem/5(HWT dem)
  TIS2_lead_velocity_[m/s]1/1 -> Stop & Go/6(Vp [m/s])
  TIS2_distance [m]1/1 -> If Action Subsystem1/4(EGO dis)
  HWT_demanded_[s]1/1 -> If Action Subsystem1/5(HWT dem)
  Stand/1 -> Stop & Go/9(Stand)
  th_in [%]1/1 -> If Action Subsystem/6(th in)
  Add2/1 -> If Action Subsystem/2(e), If Action Subsystem1/2(e)
  If Action Subsystem1/2(throttle) -> Merge1/2
  If Action Subsystem/2(throttle) -> Merge1/1
  If Action Subsystem1/1(dec) -> Merge/2
  If Action Subsystem/1(dec) -> Merge/1
  If/2 -> If Action Subsystem1/Action
  If/1 -> If Action Subsystem/Action
  EGO Velocity [m/s]1/1 -> Stop & Go/8(EGO_Velocity [m/s])
  TIS2_safe_distance [m]1/1 -> Stop & Go/5(TIS2_Safe_Distance [m])
  Stop & Go/1(BrakePres[bar]) -> TIS2_br_out [bar]/1
  Stop & Go/2(Th_out [%]) -> TIS2_th_out [%]/1
  TIS2_distance [m]3/1 -> Stop & Go/3(TIS2_Distance[m])
  Switch/1 -> Stop & Go/1(Brake_Pres_in[bar])
  th_in [%]/1 -> Switch1/3
  br_in [bar]/1 -> Switch/3
  Merge1/1 -> Switch1/1
  Gain1/1 -> Switch/1
  Switch1/1 -> Stop & Go/2(Throttle_in[%])
  TIS2_HWT_flag/1 -> TIS2_flag/1, Stop & Go/4(TIS2_HWT_flag), Switch/2, Switch1/2
  Merge/1 -> Saturation/1
  Saturation/1 -> Rate Limiter/1
  TIS2_safe_distance [m]/1 -> Add2/2
  TIS2_distance [m]/1 -> Add2/1
  Add1/1 -> If Action Subsystem/1(rd), Stop & Go/7(Rangedot [m/s]), If Action Subsystem1/1(rd)
  TIS2_lead_velocity_[m/s]/1 -> If Action Subsystem1/3(Vp), TIS2_Lead_velocity_[m/s]/1, Add1/2
  EGO Velocity [m/s]/1 -> Add1/1
  Add/1 -> If/1
  HWT_demanded_[s]/1 -> Add/2
  TIS2_HWT/1 -> TIS2_HWTo/1, Add/1

== system ACC_speed_change_curve_cs/Audi_A8_1/ACC_System3/TIS2 Bend Road ==
  note: === TIS2 Bend Road block ===
      |
      |  - interpretes information provided from the first TIS sensor,
      |  - computes HeadWay Time (HWT) for object on the lane of the EGO car on the bend road,
      |  - determines if detected objects is potentially dengerous,
      |  - outputs distance to the following car, computes its velocity and safe distance to be kept.
  EGO_velocity [m/s] : Inport
  TIS2_range [m] : Inport  Port=2  PortDimensions=TISdet(2)
  TIS2_rangedot [m/s] : Inport  Port=3  PortDimensions=TISdet(2)
  TIS2_theta [deg] : Inport  Port=4  PortDimensions=TISdet(2)
  HWT_dem [s] : Inport  Port=5
  Standstill [m] : Inport  Port=6
  EGO_Yaw_rate [deg/s] : Inport  Port=7
  EGO_velocity [m/s]2 : InportShadow
  Hold : Subsystem
  Lead Car Longitudinal Velocity : Subsystem
  TIS1 HWT Computing : Subsystem
  TIS2 Closest Object On Bend Road : Subsystem
  TIS2 HWT Flag : Subsystem
  TIS2 Objects On Bend Road : Subsystem
  TIS2 Sorting Fun : Subsystem
  TIS2_closest_object_search1 : MATLAB Function  TreatAsAtomicUnit=on
  HWT_flag : Outport
  TIS2 Lead distance [m] : Outport  Port=2
  TIS2 Safe_distance [m] : Outport  Port=3
  TIS2_HWT_bend : Outport  Port=4
  TIS2 Lead velocity [m/s] : Outport  Port=5
  index : Outport  Port=6
  wires:
  TIS2 HWT Flag/1(HWT_flag) -> Hold/1(HWTflagIN)
  Hold/1(HWT_flag) -> HWT_flag/1
  Lead Car Longitudinal Velocity/2(Lead velocity [m/s]) -> Hold/2(lead_vel_in), TIS2 Lead velocity [m/s]/1
  Lead Car Longitudinal Velocity/1(Safe distance [m]) -> TIS2 Safe_distance [m]/1
  TIS2 Closest Object On Bend Road/4(range [m]) -> Lead Car Longitudinal Velocity/7(TIS2 Range [m])
  TIS2 Closest Object On Bend Road/2(theta [rad]) -> Lead Car Longitudinal Velocity/5(theta [rad])
  TIS2 Closest Object On Bend Road/5(lambda [rad]) -> Lead Car Longitudinal Velocity/6(lambda [rad])
  Standstill [m]/1 -> TIS2 HWT Flag/4(Standstill distance), Lead Car Longitudinal Velocity/4(Standstill [m])
  TIS1 HWT Computing/1(HWT [s]) -> TIS2 HWT Flag/2(HWT [s]), TIS2_HWT_bend/1
  HWT_dem [s]/1 -> TIS2 HWT Flag/3(HWT_dem [s]), Lead Car Longitudinal Velocity/1(HWT_dem (s))
  TIS2 Closest Object On Bend Road/1(rangedot [m/s]) -> Lead Car Longitudinal Velocity/2(TIS1 Rangedot [m/s])
  EGO_velocity [m/s]2/1 -> Lead Car Longitudinal Velocity/3(EGO Velocity [m/s]), TIS1 HWT Computing/2(Velocity [m/s])
  TIS2 Closest Object On Bend Road/3(Distance [m]) -> TIS1 HWT Computing/1(Distance [m]), TIS2 HWT Flag/1(Distance closest [m]), TIS2 Lead distance [m]/1
  TIS2_closest_object_search1/1(index) -> index/1, TIS2 Closest Object On Bend Road/1(index)
  EGO_velocity [m/s]/1 -> TIS2 Objects On Bend Road/4(EGO_Velocity [m/s])
  EGO_Yaw_rate [deg/s]/1 -> TIS2 Objects On Bend Road/5(EGO_Yaw_rate_[deg/s])
  TIS2 Objects On Bend Road/5(TIS2_lambda_[rad]) -> TIS2 Closest Object On Bend Road/6(TIS2_lambda [rad])
  TIS2 Objects On Bend Road/4(TIS1_Distance [m]) -> TIS2 Closest Object On Bend Road/5(TIS2_Distance [m])
  TIS2 Objects On Bend Road/3(TIS2_THETA [rad]) -> TIS2 Closest Object On Bend Road/4(TIS2_theta [rad])
  TIS2 Objects On Bend Road/2(TIS2_RANGEDOT [m/s]) -> TIS2 Closest Object On Bend Road/3(TIS2_rangedot [m])
  TIS2 Objects On Bend Road/1(TIS2_RANGE [m]) -> TIS2_closest_object_search1/1(distance), TIS2 Closest Object On Bend Road/2(TIS2_range [m])
  TIS2 Sorting Fun/3(TIS2_THETA [rad]) -> TIS2 Objects On Bend Road/3(TIS2_theta [rad])
  TIS2 Sorting Fun/2(TIS2_RANGEDOT [m/s]) -> TIS2 Objects On Bend Road/2(TIS2_rangedot [m/s])
  TIS2 Sorting Fun/1(TIS2_RANGE [m]) -> TIS2 Objects On Bend Road/1(TIS2_range [m])
  TIS2_theta [deg]/1 -> TIS2 Sorting Fun/3(TIS2theta [deg])
  TIS2_rangedot [m/s]/1 -> TIS2 Sorting Fun/2(TIS2rangedot [m/s])
  TIS2_range [m]/1 -> TIS2 Sorting Fun/1(TIS2range [m])

== system ACC_speed_change_curve_cs/Audi_A8_1/ACC_System3/TIS2 Straight Road ==
  note: === TIS2 Straight Road block ===
      |
      |  - interpretes information provided from the second TIS sensor,
      |  - computes HeadWay Time (HWT) for object on the lane in front of the EGO car,
      |  - determines if detected objects is potentially dengerous,
      |  - outputs distance to the following car, computes its velocity and safe distance to be kept.
  EGO_velocity [m/s] : Inport
  TIS2_range [m] : Inport  Port=2  PortDimensions=TISdet(2)
  TIS2_rangedot [m/s] : Inport  Port=3  PortDimensions=TISdet(2)
  TIS2_theta [deg] : Inport  Port=4  PortDimensions=TISdet(2)
  HWT_dem [s] : Inport  Port=5
  Standstill [m] : Inport  Port=6
  HWT_dem [s]1 : InportShadow  Port=5
  Hold : Subsystem
  TIS2 Closest Object : Subsystem
  TIS2 HWT Computing : Subsystem
  TIS2 HWT Computing2 : Subsystem
  TIS2 HWT Flag : Subsystem
  TIS2 Lead Car Longitudinal Velocity : Subsystem
  TIS2 Objects On Lane : Subsystem
  TIS2 Sorting Fun : Subsystem
  TIS2_closest_object_search : MATLAB Function  TreatAsAtomicUnit=on
  HWT_flag : Outport
  TIS2 Lead distance [m] : Outport  Port=2
  TIS2 Safe_distance [m] : Outport  Port=3
  TIS2_HWT_straight : Outport  Port=4
  TIS2 Lead velocity [m/s] : Outport  Port=5
  index : Outport  Port=6
  wires:
  TIS2 Objects On Lane/2(TIS2_Distance [m]) -> TIS2 HWT Computing/1(Distance [m]), TIS2_closest_object_search/1(distance), TIS2 Closest Object/2(TIS2_distance [m])
  HWT_dem [s]1/1 -> TIS2 HWT Computing/2(HWT demanded)
  Hold/1(HWT_flag) -> HWT_flag/1
  TIS2 HWT Flag/1(HWT_flag) -> Hold/1(HWTflagIN)
  TIS2 HWT Computing2/1(HWT [s]) -> TIS2_HWT_straight/1
  TIS2 Lead Car Longitudinal Velocity/2(Lead velocity [m/s]) -> Hold/2(lead_vel_in), TIS2 Lead velocity [m/s]/1
  TIS2 Objects On Lane/1(TIS2_RANGEDOT [m/s]) -> TIS2 Closest Object/1(TIS2_rangedot [m/s])
  Standstill [m]/1 -> TIS2 HWT Flag/4(Standstill distance), TIS2 Lead Car Longitudinal Velocity/4(Standstill [m])
  TIS2_range [m]/1 -> TIS2 Sorting Fun/1(TIS2range [m])
  TIS2_rangedot [m/s]/1 -> TIS2 Sorting Fun/2(TIS2rangedot [m/s])
  TIS2_theta [deg]/1 -> TIS2 Sorting Fun/3(TIS2theta [deg])
  TIS2 Sorting Fun/1(TIS2_RANGE [m]) -> TIS2 Objects On Lane/1(TIS2_range [m])
  TIS2 Sorting Fun/2(TIS2_RANGEDOT [m/s]) -> TIS2 Objects On Lane/2(TIS2_rangedot [m/s])
  TIS2 Sorting Fun/3(TIS2_THETA [rad]) -> TIS2 Objects On Lane/3(TIS2_theta [rad])
  TIS2_closest_object_search/1(index) -> index/1, TIS2 Closest Object/3(index)
  TIS2 HWT Computing/1(HWT [s]) -> TIS2 HWT Flag/3(HWT [s])
  EGO_velocity [m/s]/1 -> TIS2 HWT Computing/3(Velocity [m/s]), TIS2 HWT Computing2/2(Velocity [m/s]), TIS2 Lead Car Longitudinal Velocity/3(EGO Velocity [m/s])
  TIS2 Closest Object/2(distance [m/s]) -> TIS2 HWT Flag/1(Distance closest [m]), TIS2 HWT Computing2/1(Distance [m]), TIS2 Lead distance [m]/1
  TIS2 Closest Object/1(rangedot [m/s]) -> TIS2 Lead Car Longitudinal Velocity/2(TIS2 Rangedot [m/s])
  HWT_dem [s]/1 -> TIS2 HWT Flag/2(HWT_dem [s]), TIS2 Lead Car Longitudinal Velocity/1(HWT_dem (s))
  TIS2 Lead Car Longitudinal Velocity/1(Safe distance [m]) -> TIS2 Safe_distance [m]/1

== system ACC_speed_change_curve_cs/Audi_A8_1/CarSim2PreScan/Transformation_SprungMassdSPACE2PreScan ==
  In1 : Inport
  Demux : Demux  Outputs=3
  Ini z-position VEHICLE wrt GLOBAL axis system [m] : Constant  Value=z0
  Mux : Mux  Inputs=3
  Sum1 : Sum  Inputs=+-
  Out1 : Outport
  wires:
  Mux/1 -> Out1/1
  Ini z-position VEHICLE wrt GLOBAL axis system [m]/1 -> Sum1/2
  Demux/1 -> Mux/1
  Sum1/1 -> Mux/3
  Demux/3 -> Sum1/1
  Demux/2 -> Mux/2
  In1/1 -> Demux/1

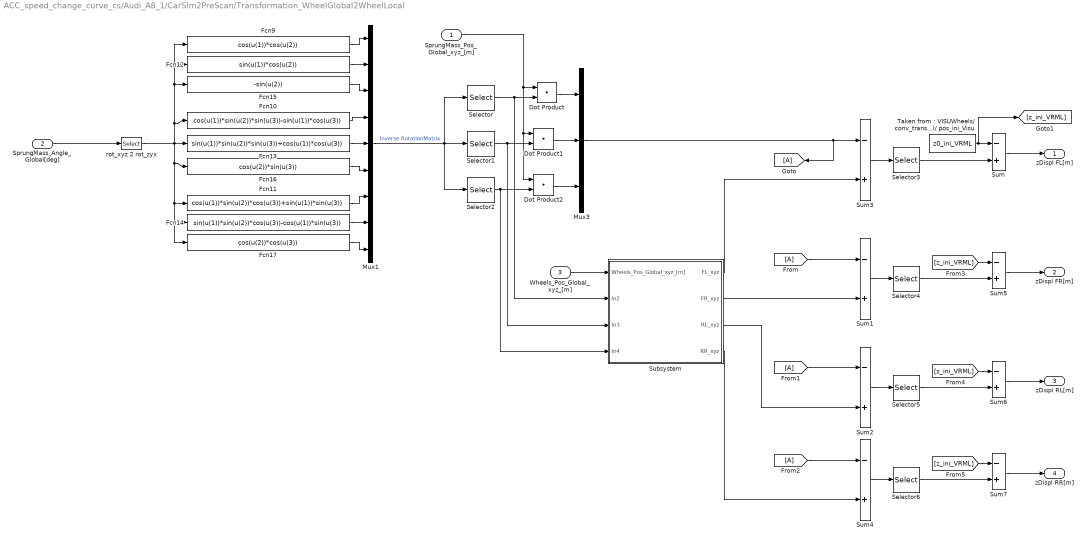
== system ACC_speed_change_curve_cs/Audi_A8_1/CarSim2PreScan/Transformation_WheelGlobal2WheelLocal ==
  SprungMass_Pos_Global_xyz_[m] : Inport
  SprungMass_Angle_Global[deg] : Inport  Port=2
  Wheels_Pos_Global_xyz_[m] : Inport  Port=3
  Dot Product : DotProduct  InputSameDT=on  OutDataTypeStr=Inherit: Inherit via internal rule
  Dot Product1 : DotProduct  InputSameDT=on  OutDataTypeStr=Inherit: Inherit via internal rule
  Dot Product2 : DotProduct  InputSameDT=on  OutDataTypeStr=Inherit: Inherit via internal rule
  Fcn10 : Fcn  Expr=cos(u(1))*sin(u(2))*sin(u(3))-sin(u(1))*cos(u(3))
  Fcn11 : Fcn  Expr=cos(u(1))*sin(u(2))*cos(u(3))+sin(u(1))*sin(u(3))
  Fcn12 : Fcn  Expr=sin(u(1))*cos(u(2))
  Fcn13 : Fcn  Expr=sin(u(1))*sin(u(2))*sin(u(3))+cos(u(1))*cos(u(3))
  Fcn14 : Fcn  Expr=sin(u(1))*sin(u(2))*cos(u(3))-cos(u(1))*sin(u(3))
  Fcn15 : Fcn  Expr=-sin(u(2))
  Fcn16 : Fcn  Expr=cos(u(2))*sin(u(3))
  Fcn17 : Fcn  Expr=cos(u(2))*cos(u(3))
  Fcn9 : Fcn  Expr=cos(u(1))*cos(u(2))
  Mux1 : Mux  Inputs=9
  Mux3 : Mux  Inputs=3
  Selector : Selector  InputPortWidth=9  IndexOptions=Index vector (dialog)  Indices=[1 2 3]  OutputSizes=1
  Selector1 : Selector  InputPortWidth=9  IndexOptions=Index vector (dialog)  Indices=[4 5 6]  OutputSizes=1
  Selector2 : Selector  InputPortWidth=9  IndexOptions=Index vector (dialog)  Indices=[7 8 9]  OutputSizes=1
  Selector{3..6} (4 alike) : Selector  InputPortWidth=3  IndexOptions=Index vector (dialog)  Indices=[3]  OutputSizes=1
  Subsystem : Subsystem
  Sum{,1..7} (8 alike) : Sum  Inputs=-+
  "Taken from : VISUWheels/ conv_transWheel/ pos_ini_Visu" : Constant  Value=z0_ini_VRML
  rot_xyz 2 rot_zyx : Selector  InputPortWidth=3  IndexOptions=Index vector (dialog)  Indices=[3 2 1]  OutputSizes=1
  zDispl FL[m] : Outport
  zDispl FR[m] : Outport  Port=2
  zDispl RL[m] : Outport  Port=3
  zDispl RR[m] : Outport  Port=4
  wires:
  "Taken from : VISUWheels/ conv_transWheel/ pos_ini_Visu"/1 -> [z_ini_VRML], Sum/1
  [z_ini_VRML] -> Sum7/1
  [z_ini_VRML] -> Sum6/1
  [z_ini_VRML] -> Sum5/1
  [A] -> Sum4/1
  [A] -> Sum2/1
  [A] -> Sum1/1
  Sum4/1 -> Selector6/1
  Selector6/1 -> Sum7/2
  Sum7/1 -> zDispl RR[m]/1
  Sum2/1 -> Selector5/1
  Selector5/1 -> Sum6/2
  Sum6/1 -> zDispl RL[m]/1
  Sum1/1 -> Selector4/1
  Selector4/1 -> Sum5/2
  Sum5/1 -> zDispl FR[m]/1
  Subsystem/4(RR_xyz) -> Sum4/2
  Subsystem/3(RL_xyz) -> Sum2/2
  Subsystem/2(FR_xyz) -> Sum1/2
  Selector3/1 -> Sum/2
  Sum/1 -> zDispl FL[m]/1
  Subsystem/1(FL_xyz) -> Sum3/2
  Wheels_Pos_Global_xyz_[m]/1 -> Subsystem/1(Wheels_Pos_Global_xyz_[m])
  Sum3/1 -> Selector3/1
  SprungMass_Angle_Global[deg]/1 -> rot_xyz 2 rot_zyx/1
  Mux3/1 -> [A], Sum3/1
  rot_xyz 2 rot_zyx/1 -> Fcn16/1, Fcn11/1, Fcn14/1, Fcn17/1, Fcn13/1, Fcn10/1, Fcn15/1, Fcn12/1, Fcn9/1
  Dot Product1/1 -> Mux3/2
  Dot Product2/1 -> Mux3/3
  Selector2/1 -> Subsystem/4(In4), Dot Product2/2
  Selector1/1 -> Subsystem/3(In3), Dot Product1/2
  Dot Product/1 -> Mux3/1
  SprungMass_Pos_Global_xyz_[m]/1 -> Dot Product/1, Dot Product2/1, Dot Product1/1
  Selector/1 -> Subsystem/2(In2), Dot Product/2
  Mux1/1 -> Selector2/1, Selector1/1, Selector/1  "Inverse RotationMatrix"
  Fcn17/1 -> Mux1/9
  Fcn14/1 -> Mux1/8
  Fcn11/1 -> Mux1/7
  Fcn16/1 -> Mux1/6
  Fcn13/1 -> Mux1/5
  Fcn10/1 -> Mux1/4
  Fcn15/1 -> Mux1/3
  Fcn12/1 -> Mux1/2
  Fcn9/1 -> Mux1/1

== system ACC_speed_change_curve_cs/Audi_A8_1/PathFollower_1/CTRL REFERENCES ==
  note: REFERENCE POSITION BASED POSITION CTRL
  Pos x,y,Y [m,m,rad] : Inport
  Position Preview Distance [m] : Inport  Port=2
  TrajOffset [m,m,rad] : Inport  Port=3
  ActorOffset_Left(+) / Right(-)_[m] : Inport  Port=4
  Calculate Preview Point (pvp) by extrapolating current Vehicle Position (p0) with Preview Distance and Vehicle Orientation : Subsystem
  Demux : Demux  Outputs=[2 2]
  Demux1 : Demux  Outputs=2
  Demux2 : Demux  Outputs=2
  Find Reference Point (pref) on Trajectory closest to PVP Point (pvp) : Subsystem
      mask Display:
      | port_label('input',1,'pvp [m,m]');
      | port_label('input',2,'TrajOffset_x_y_Y [m,m,rad]');
      | port_label('input',3,'ActorOffset_Left_Right [m]');
      | port_label('input',4,'p0 [m,m,rad]');
      | port_label('output',1,'pref [m,m]');
      | port_label('output',2,'Actor_traj_distance [m]');
      | port_label('output',3,'Actor_traj_angle [m]');
  Mux1 : Mux  Inputs=2
  Reshape : Reshape  OutputDimensionality=Customize  OutputDimensions=[2,2]
  Selector1 : Selector  InputPortWidth=3  IndexOptions=Index vector (dialog)  Indices=[1 2]  OutputSizes=1
  Terminator : Terminator
  Terminator1 : Terminator
  Terminator2 : Terminator
  Vector Concatenate : Concatenate
  pvp  [m,m] : Outport
  pref_pvp [m,m] : Outport  Port=2
  pref_0 [m,m] : Outport  Port=3
  Actor/Traj_distance [m] : Outport  Port=4
  Actor/Traj_angle [deg] : Outport  Port=5
  wires:
  Demux1/2 -> Terminator2/1
  Demux2/2 -> Terminator1/1
  Demux1/1 -> Actor/Traj_distance [m]/1
  Demux2/1 -> Actor/Traj_angle [deg]/1
  Find Reference Point (pref) on Trajectory closest to PVP Point (pvp)/1(Out1) -> Demux/1
  Reshape/1 -> Find Reference Point (pref) on Trajectory closest to PVP Point (pvp)/1(In1)
  Vector Concatenate/1 -> Reshape/1
  Mux1/1 -> Vector Concatenate/2, pvp  [m,m]/1
  Pos x,y,Y [m,m,rad]/1 -> Calculate Preview Point (pvp) by extrapolating current Vehicle Position (p0) with Preview Distance and Vehicle Orientation/2(x,y,Y Demux [m,m,rad]), Find Reference Point (pref) on Trajectory closest to PVP Point (pvp)/4(In4), Selector1/1
  Calculate Preview Point (pvp) by extrapolating current Vehicle Position (p0) with Preview Distance and Vehicle Orientation/1(x_glob_PVD) -> Mux1/1
  Calculate Preview Point (pvp) by extrapolating current Vehicle Position (p0) with Preview Distance and Vehicle Orientation/3(Y [rad]) -> Terminator/1
  Position Preview Distance [m]/1 -> Calculate Preview Point (pvp) by extrapolating current Vehicle Position (p0) with Preview Distance and Vehicle Orientation/1(Preview Distance)
  Demux/2 -> pref_pvp [m,m]/1
  Demux/1 -> pref_0 [m,m]/1
  Calculate Preview Point (pvp) by extrapolating current Vehicle Position (p0) with Preview Distance and Vehicle Orientation/2(y_glob_PVD) -> Mux1/2
  TrajOffset [m,m,rad]/1 -> Find Reference Point (pref) on Trajectory closest to PVP Point (pvp)/2(In2)  "L6"
  ActorOffset_Left(+) / Right(-)_[m]/1 -> Find Reference Point (pref) on Trajectory closest to PVP Point (pvp)/3(In3)
  Selector1/1 -> Vector Concatenate/1
  Find Reference Point (pref) on Trajectory closest to PVP Point (pvp)/2(Out2) -> Demux1/1
  Find Reference Point (pref) on Trajectory closest to PVP Point (pvp)/3(Out3) -> Demux2/1

== system ACC_speed_change_curve_cs/Audi_A8_1/PathFollower_1/Calculate shifted p0 wrt COG ==
  position x,y,Y [m,m,deg] : Inport
  Constant1 : Constant  Value=XShifting_wrt_COG
  Degrees to Radians : simulink_extras/Transformations/Degrees to Radians
  Demux1 : Demux  Outputs=3
  Fcn : Fcn  Expr=u(2)*cos(u(1))
  Fcn1 : Fcn  Expr=u(2)*sin(u(1))
  Mux1 : Mux  Inputs=3
  Mux2 : Mux  Inputs=2
  Sum : Sum  Inputs=|++
  Sum1 : Sum  Inputs=|++
  position x,y,Y [m,m,rad] : Outport
  wires:
  Sum/1 -> Mux1/1
  Sum1/1 -> Mux1/2
  Demux1/1 -> Sum/1
  Demux1/3 -> Degrees to Radians/1
  Degrees to Radians/1 -> Mux2/1, Mux1/3
  Mux2/1 -> Fcn/1, Fcn1/1
  Fcn/1 -> Sum/2
  Fcn1/1 -> Sum1/2
  Demux1/2 -> Sum1/1
  position x,y,Y [m,m,deg]/1 -> Demux1/1
  Mux1/1 -> position x,y,Y [m,m,rad]/1
  Constant1/1 -> Mux2/2
